simulink model "TVC6DofFins"  (R2024b)
settings: Solver=VariableStepAuto  StartTime=0.0  StopTime=10.0  RelTol=1e-3
libraries: shared6dof x1
settings Model: Creator=jebid  LastModifiedBy=jebid

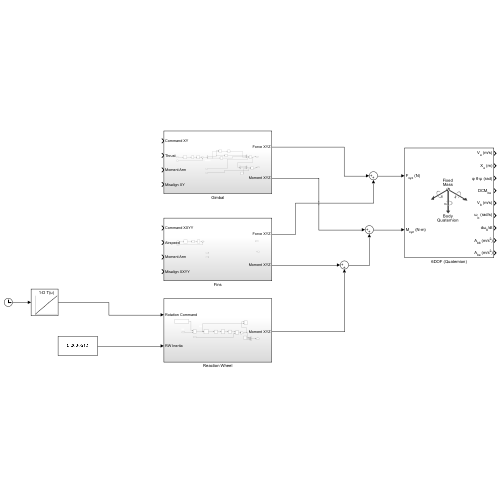
[thumbnail: Simulink's stored preview of the top-level diagram]
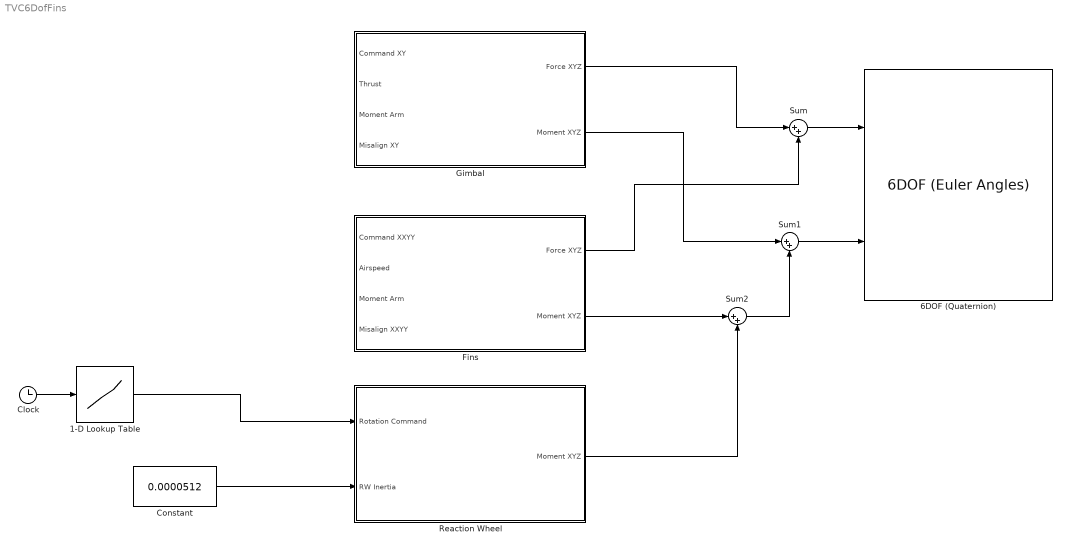
== system TVC6DofFins ==
  1-D Lookup Table : Lookup_n-D  NumberOfTableDimensions=1  BreakpointsForDimension1=[0;2;4;6;8;10]  Table=[0;800;1600;2400;3200;4000]  InternalRulePriority=Speed  RndMeth=Simplest
  6DOF (Quaternion) : shared6dof/6DOF (Euler Angles)  units=Metric (MKS)  mtype=Fixed  rep=Quaternion  xme_0=[0 0 0]  Vm_0=[0 0 0]  eul_0=[0 0 0]  pm_0=[0 0 0]  mass_0=1.0  mass_e=0.5  mass_f=2.0  inertia=[0.083694 0 0; 0 0.083694 0; 0 0 0.000722]  inertia_e=eye(3)  inertia_f=2*eye(3)  k_quat=1.0  vre_flag=on  abi_flag=on  aMode=0  xme_statename=''  Vm_statename=''  eul_statename=''  quat_statename=''  pm_statename=''  mass_statename=''
      settings: LibrarySourceBlock=aerolib6dof2/6DOF (Quaternion)
  Clock : Clock
  Constant : Constant  Value=0.0000512
  Fins : Subsystem
  Gimbal : Subsystem
  Reaction Wheel : Subsystem
  Sum : Sum  Inputs=|++
  Sum1 : Sum  Inputs=|++
  Sum2 : Sum  Inputs=|++
  wires:
  Sum/1 -> 6DOF (Quaternion)/1
  Sum1/1 -> 6DOF (Quaternion)/2
  Gimbal/2(Moment XYZ) -> Sum1/1
  Gimbal/1(Force XYZ) -> Sum/1
  Fins/1(Force XYZ) -> Sum/2
  Fins/2(Moment XYZ) -> Sum2/1
  Sum2/1 -> Sum1/2
  Reaction Wheel/1(Moment XYZ) -> Sum2/2
  Constant/1 -> Reaction Wheel/2(RW Inertia)
  1-D Lookup Table/1 -> Reaction Wheel/1(Rotation Command)
  Clock/1 -> 1-D Lookup Table/1

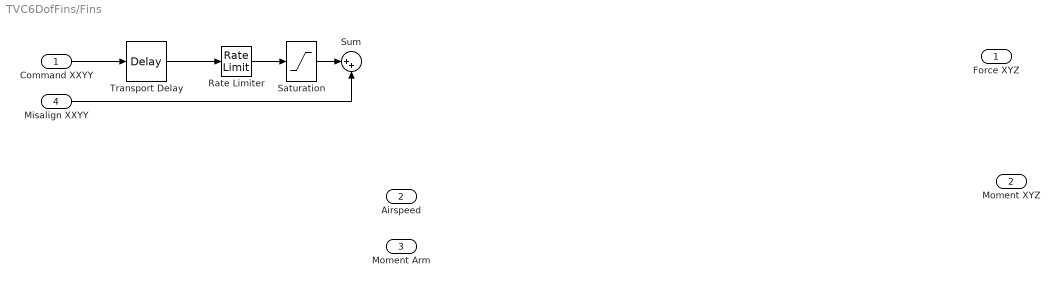
== system TVC6DofFins/Fins ==
  Command XXYY : Inport  PortDimensions=4
  Airspeed : Inport  Port=2  PortDimensions=1
  Moment Arm : Inport  Port=3  PortDimensions=1
  Misalign XXYY : Inport  Port=4  PortDimensions=4
  Rate Limiter : RateLimiter  RisingSlewLimit=0.9  FallingSlewLimit=-0.9
  Saturation : Saturate  UpperLimit=0.0872665  LowerLimit=-0.0872665
  Sum : Sum  Inputs=|++
  Transport Delay : TransportDelay  DelayTime=0.03
  Force XYZ : Outport  PortDimensions=3
  Moment XYZ : Outport  Port=2  PortDimensions=3
  wires:
  Command XXYY/1 -> Transport Delay/1
  Misalign XXYY/1 -> Sum/2
  Saturation/1 -> Sum/1
  Rate Limiter/1 -> Saturation/1
  Transport Delay/1 -> Rate Limiter/1

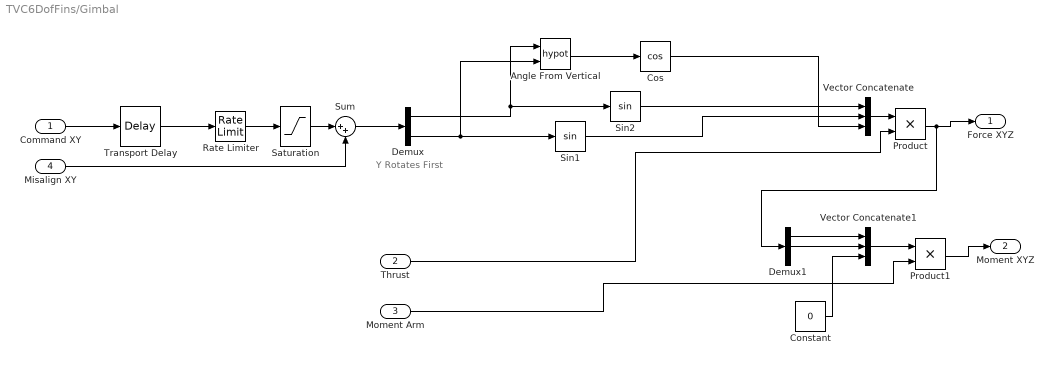
== system TVC6DofFins/Gimbal ==
  note: Y Rotates First
  Command XY : Inport  PortDimensions=2
  Thrust : Inport  Port=2  PortDimensions=1
  Moment Arm : Inport  Port=3  PortDimensions=1
  Misalign XY : Inport  Port=4  PortDimensions=2
  Angle From Vertical : Math  Operator=hypot
  Constant : Constant  Value=0
  Cos : Trigonometry  Operator=cos
  Demux : Demux  Outputs=2
  Demux1 : Demux  Outputs=3
  Product : Product
  Product1 : Product
  Rate Limiter : RateLimiter  RisingSlewLimit=0.9  FallingSlewLimit=-0.9
  Saturation : Saturate  UpperLimit=0.0872665  LowerLimit=-0.0872665
  Sin1 : Trigonometry
  Sin2 : Trigonometry
  Sum : Sum  Inputs=|++
  Transport Delay : TransportDelay  DelayTime=0.03
  Vector Concatenate : Concatenate  NumInputs=3
  Vector Concatenate1 : Concatenate  NumInputs=3
  Force XYZ : Outport  PortDimensions=3
  Moment XYZ : Outport  Port=2  PortDimensions=3
  wires:
  Demux/1 -> Sin2/1, Angle From Vertical/1
  Demux/2 -> Sin1/1, Angle From Vertical/2
  Cos/1 -> Vector Concatenate/3
  Angle From Vertical/1 -> Cos/1
  Vector Concatenate/1 -> Product/1
  Constant/1 -> Vector Concatenate1/3
  Command XY/1 -> Transport Delay/1
  Misalign XY/1 -> Sum/2
  Sum/1 -> Demux/1
  Saturation/1 -> Sum/1
  Rate Limiter/1 -> Saturation/1
  Transport Delay/1 -> Rate Limiter/1
  Product/1 -> Demux1/1, Force XYZ/1
  Thrust/1 -> Product/2
  Demux1/2 -> Vector Concatenate1/2
  Demux1/1 -> Vector Concatenate1/1
  Vector Concatenate1/1 -> Product1/1
  Product1/1 -> Moment XYZ/1
  Moment Arm/1 -> Product1/2
  Sin1/1 -> Vector Concatenate/2
  Sin2/1 -> Vector Concatenate/1

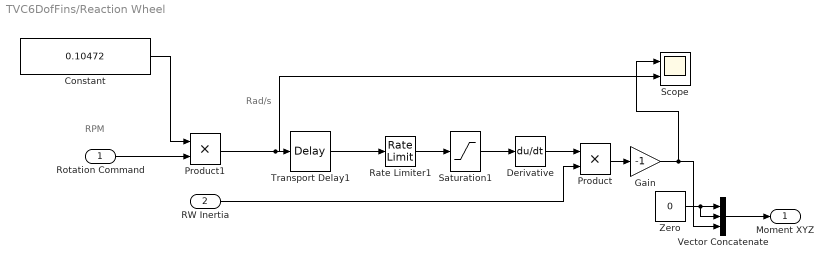
== system TVC6DofFins/Reaction Wheel ==
  note: Rad/s
  note: RPM
  Rotation Command : Inport  PortDimensions=1
  RW Inertia : Inport  Port=2  PortDimensions=1
  Constant : Constant  Value=0.10472
  Derivative : Derivative
  Gain : Gain  Gain=-1
  Product : Product
  Product1 : Product
  Rate Limiter1 : RateLimiter  RisingSlewLimit=1000  FallingSlewLimit=-1000
  Saturation1 : Saturate  UpperLimit=4200  LowerLimit=-4200
  Scope : Scope  NumInputPorts=2
  Transport Delay1 : TransportDelay  DelayTime=0.03
  Vector Concatenate : Concatenate  NumInputs=3
  Zero : Constant  Value=0  OutDataTypeStr=Inherit: Inherit via back propagation
  Moment XYZ : Outport  PortDimensions=3
  wires:
  Transport Delay1/1 -> Rate Limiter1/1
  Rate Limiter1/1 -> Saturation1/1
  RW Inertia/1 -> Product/2
  Vector Concatenate/1 -> Moment XYZ/1
  Zero/1 -> Vector Concatenate/2, Vector Concatenate/1
  Saturation1/1 -> Derivative/1
  Derivative/1 -> Product/1
  Product/1 -> Gain/1
  Rotation Command/1 -> Product1/2
  Product1/1 -> Scope/2, Transport Delay1/1
  Constant/1 -> Product1/1
  Gain/1 -> Scope/1, Vector Concatenate/3
